simulink model "Koopman_nlMPC"  (R2022b)
settings: Solver=FixedStepAuto  StartTime=0.0  StopTime=Tf  FixedStep=Ts  RelTol=1e-3
values from neighbouring files (symbols this model uses):
  A_EKF = A(1:n_x,:)    [vdp_MPC.m]
  B_EKF = B(1:n_x,:)    [vdp_MPC.m]
  C_EKF = C    [vdp_MPC.m]
  D = zeros(size(X,1),n_u)    [EKF_Koopman.m]
  eta = 0.001    [vdp_MPC.m]
  S0_EKF = Spline_Radial_Obs([0;0], X0)    [vdp_MPC.m]
  Ts = 0.01    [EKF_Koopman.m]    (also in scope_plotting.m)
undefined symbols (not defined in the file or in its folder): DiscIntNeverNeededParam
libraries: mpclib x1
settings Model: Creator=sergiovaneg  LastModifiedBy=sergiovaneg
settings ModelReferenceCC: EnableRefExpFcnMdlSchedulingChecks=on

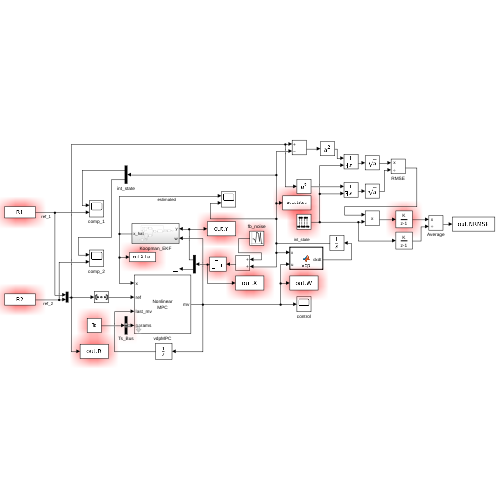
[thumbnail: Simulink's stored preview of the top-level diagram]
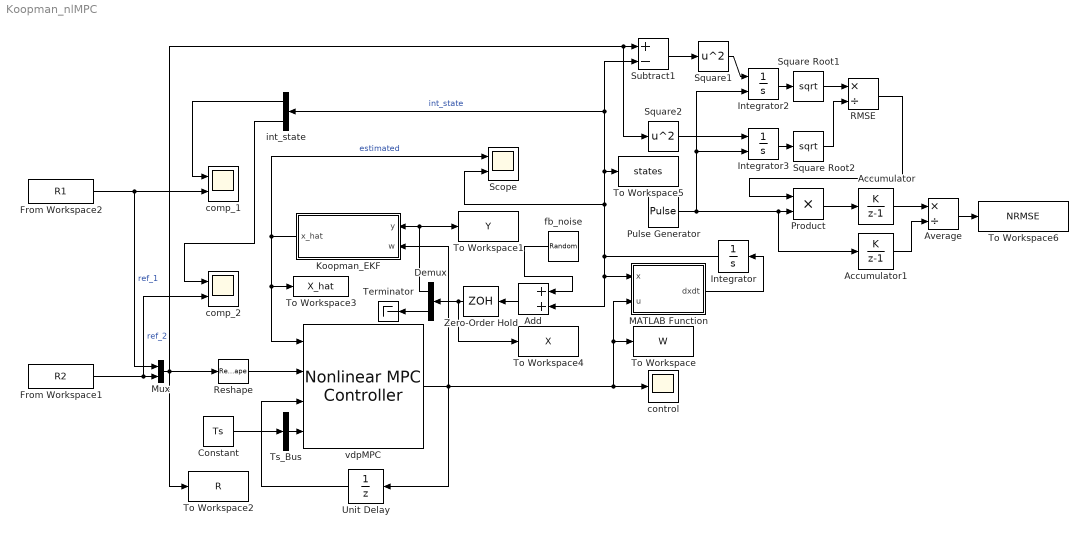
== system Koopman_nlMPC ==
  Accumulator : DiscreteIntegrator  IntegratorMethod=Accumulation: Forward Euler  InitialCondition=[0;0]  SampleTime=Ts  ICPrevOutput=DiscIntNeverNeededParam  ICPrevScaledInput=DiscIntNeverNeededParam
  Accumulator1 : DiscreteIntegrator  IntegratorMethod=Accumulation: Forward Euler  SampleTime=-1  ICPrevOutput=DiscIntNeverNeededParam  ICPrevScaledInput=DiscIntNeverNeededParam
  Add : Sum
  Average : Product  Inputs=*/
  Constant : Constant  Value=Ts
  Demux : Demux  Outputs=2
  From Workspace1 : FromWorkspace  VariableName=R2
  From Workspace2 : FromWorkspace  VariableName=R1
  Integrator : Integrator  InitialCondition=[0;0]
  Integrator2 : Integrator  ExternalReset=falling  InitialCondition=[0;0]
  Integrator3 : Integrator  ExternalReset=falling  InitialCondition=[eps;eps]
  Koopman_EKF : Subsystem
  MATLAB Function : MATLAB Function  TreatAsAtomicUnit=on
  Mux : Mux  Inputs=2
  Product : Product
  Pulse Generator : DiscretePulseGenerator  Period=10/Ts  SampleTime=Ts
  RMSE : Product  Inputs=*/
  Reshape : Reshape  OutputDimensionality=Row vector (2-D)
  Scope : Scope  NumInputPorts=2
  Square Root1 : Sqrt
  Square Root2 : Sqrt
  Square1 : Math  Operator=square
  Square2 : Math  Operator=square
  Subtract1 : Sum  Inputs=+-
  Terminator : Terminator
  To Workspace : ToWorkspace  VariableName=W  SampleTime=Ts
      settings: Save2DSignal=2-D array (concatenate along first dimension)
  To Workspace1 : ToWorkspace  VariableName=Y  SampleTime=Ts
      settings: Save2DSignal=2-D array (concatenate along first dimension)
  To Workspace2 : ToWorkspace  VariableName=R  SampleTime=Ts
      settings: Save2DSignal=2-D array (concatenate along first dimension)
  To Workspace3 : ToWorkspace  VariableName=X_hat  SampleTime=Ts
      settings: Save2DSignal=2-D array (concatenate along first dimension)
  To Workspace4 : ToWorkspace  VariableName=X  SampleTime=Ts
      settings: Save2DSignal=2-D array (concatenate along first dimension)
  To Workspace5 : ToWorkspace  VariableName=states  SampleTime=Ts
      settings: Save2DSignal=2-D array (concatenate along first dimension)
  To Workspace6 : ToWorkspace  VariableName=NRMSE  SampleTime=-1
      settings: MaxDataPoints=1  Save2DSignal=2-D array (concatenate along first dimension)
  Ts_Bus : BusCreator  Inputs=1  OutDataTypeStr=Bus: Ts_Bus_1  NonVirtualBus=on
      settings: InheritFromInputs=off
  Unit Delay : UnitDelay  SampleTime=-1  HasFrameUpgradeWarning=on
  Zero-Order Hold : ZeroOrderHold  SampleTime=Ts
  comp_1 : Scope  NumInputPorts=2
  comp_2 : Scope  NumInputPorts=2
  control : Scope
  fb_noise : RandomNumber  Variance=eta  Seed=[2;3]  SampleTime=Ts
  int_state : Demux  Outputs=2
  vdpMPC : mpclib/Nonlinear MPC Controller  nlmpcobj=nlobj  UseObjectTs=on  UseMEX=off  md_enabled=off  mvtarget_enabled=off  param_enabled=on  cost_enabled=off  mvseq_enabled=off  stateseq_enabled=off  ovseq_enabled=off  slack_enabled=off  status_enabled=off  ov_min=off  ov_max=off  mv_min=off  mv_max=off  mvrate_min=off  mvrate_max=off  state_min=off  state_max=off  ov_weight=off  mv_weight=off  mvrate_weight=off  ecr_weight=off  nlp_initialize=off
  wires:
  int_state/1 -> comp_1/1
  fb_noise/1 -> Add/1
  Reshape/1 -> vdpMPC/2
  vdpMPC/1 -> Koopman_EKF/2(w), MATLAB Function/2(u), To Workspace/1, control/1, Unit Delay/1
  Constant/1 -> Ts_Bus/1
  Integrator/1 -> To Workspace5/1, Subtract1/2, int_state/1, Scope/2, Add/2, MATLAB Function/1(x)  "int_state"
  From Workspace1/1 -> comp_2/2, Mux/2  "ref_2"
  Unit Delay/1 -> vdpMPC/3
  int_state/2 -> comp_2/1
  MATLAB Function/1(dxdt) -> Integrator/1
  Mux/1 -> Square2/1, Subtract1/1, To Workspace2/1, Reshape/1
  Ts_Bus/1 -> vdpMPC/4
  Demux/1 -> Koopman_EKF/1(y), To Workspace1/1
  Demux/2 -> Terminator/1
  Koopman_EKF/1(x_hat) -> Scope/1, vdpMPC/1, To Workspace3/1  "estimated"
  Zero-Order Hold/1 -> To Workspace4/1, Demux/1
  Add/1 -> Zero-Order Hold/1
  From Workspace2/1 -> comp_1/2, Mux/1  "ref_1"
  Square Root2/1 -> RMSE/2
  Product/1 -> Accumulator/1
  Integrator3/1 -> Square Root2/1
  Accumulator/1 -> Average/1
  RMSE/1 -> Product/1
  Accumulator1/1 -> Average/2
  Average/1 -> To Workspace6/1
  Square2/1 -> Integrator3/1
  Square Root1/1 -> RMSE/1
  Integrator2/1 -> Square Root1/1
  Square1/1 -> Integrator2/1
  Pulse Generator/1 -> Integrator2/2, Integrator3/2, Accumulator1/1, Product/2
  Subtract1/1 -> Square1/1

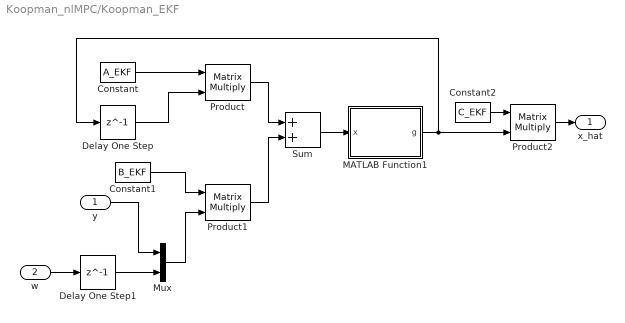
== system Koopman_nlMPC/Koopman_EKF ==
  y : Inport
  w : Inport  Port=2
  Constant : Constant  Value=A_EKF
  Constant1 : Constant  Value=B_EKF
  Constant2 : Constant  Value=C_EKF
  Delay One Step : Delay  DelayLength=1  InitialCondition=S0_EKF
  Delay One Step1 : Delay  DelayLength=1  InitialCondition=0
  MATLAB Function1 : MATLAB Function  TreatAsAtomicUnit=on
  Mux : Mux  Inputs=2
  Product : Product  Multiplication=Matrix(*)
  Product1 : Product  Multiplication=Matrix(*)
  Product2 : Product  Multiplication=Matrix(*)
  Sum : Sum
  x_hat : Outport
  wires:
  Constant/1 -> Product/1
  Delay One Step/1 -> Product/2
  Product/1 -> Sum/1
  Constant1/1 -> Product1/1
  Product1/1 -> Sum/2
  Sum/1 -> MATLAB Function1/1(x)
  Constant2/1 -> Product2/1
  Product2/1 -> x_hat/1
  w/1 -> Delay One Step1/1
  y/1 -> Mux/1
  Mux/1 -> Product1/2
  Delay One Step1/1 -> Mux/2
  MATLAB Function1/1(g) -> Product2/2, Delay One Step/1

== matlab function Koopman_nlMPC/Koopman_EKF/MATLAB Function1 ==
  data: x input; g output; X0_EKF parameter
function g = observe(x,X0_EKF)
    g=zeros(size(x,1)+size(X0_EKF,2),1);
    aux = vecnorm(X0_EKF-x)';
    g(1:size(x,1))=x;
    g(size(x,1)+1:end)=aux.*log(aux.^aux);
end

== matlab function Koopman_nlMPC/MATLAB Function ==
  data: x input; u input; dxdt output
function dxdt = vdp(x,u)
    dxdt = zeros(2,1);
    dxdt(1) = 2*x(2);
    dxdt(2) = -0.8*x(1)+2*x(2)-10*(x(1)^2)*x(2)+u;
